simulink model "EstudioReguladores"  (R2024b)
settings: Solver=VariableStepAuto  StartTime=0.0  StopTime=50000  RelTol=1e-3
undefined symbols (not defined in the file): n, p1, p2, p3, Vi
libraries: slpidlib x32
(part 3 of 4)

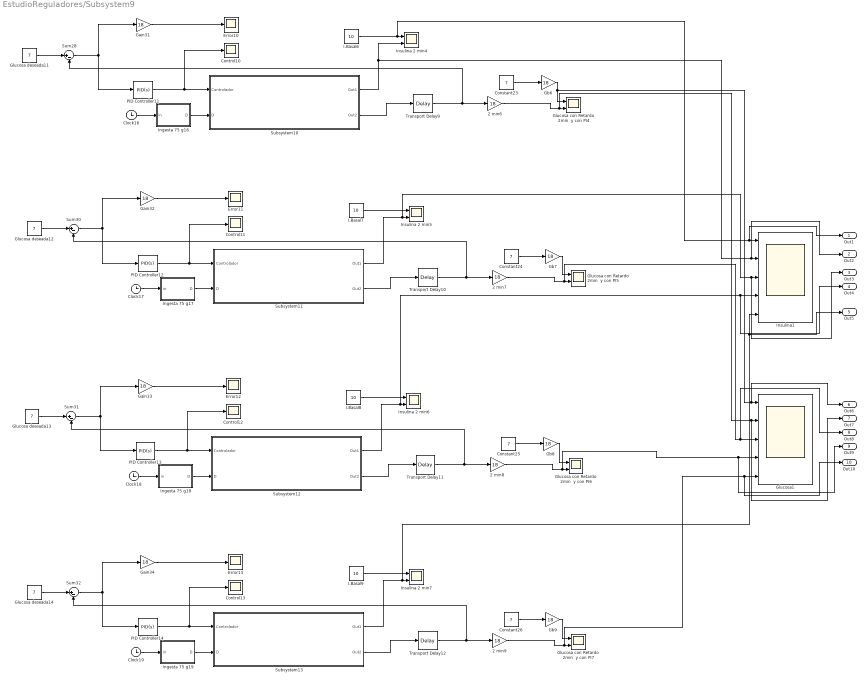
== system EstudioReguladores/Subsystem9 ==
  2 min{6..9} (4 alike) : Gain  Gain=18
  Clock{16..19} (4 alike) : Clock
  Constant{23..26} (4 alike) : Constant  Value=7
  Control{10..13} (4 alike) : Scope
  Error{10..13} (4 alike) : Scope
  Gain{31..34} (4 alike) : Gain  Gain=18
  Gb{6..9} (4 alike) : Gain  Gain=18
  Glucosa con Retardo 2min  y con PI{4..7} (4 alike) : Scope  NumInputPorts=2
  Glucosa deseada{11..14} (4 alike) : Constant  Value=7
  Glucosa1 : Scope  NumInputPorts=5
  I.Basal{6..9} (4 alike) : Constant  Value=10
  Ingesta 75 g16 : MATLAB Function  TreatAsAtomicUnit=on
  Ingesta 75 g17 : MATLAB Function  TreatAsAtomicUnit=on
  Ingesta 75 g18 : MATLAB Function  TreatAsAtomicUnit=on
  Ingesta 75 g19 : MATLAB Function  TreatAsAtomicUnit=on
  Insulina 2 min{4..7} (4 alike) : Scope  NumInputPorts=2
  Insulina1 : Scope  NumInputPorts=5
  PID Controller11 : slpidlib/PID Controller  Controller=PID  Form=Parallel  TimeDomain=Continuous-time  UseExternalTs=off  SampleTime=-1  IntegratorMethod=Forward Euler  FilterMethod=Forward Euler  ControllerParametersSource=internal  P=-0.3195  I=-0.3195/2998.95  UseKiTs=off  D=0  UseExternalDerivativeSource=off  N=10  UseFilter=on  TunerSelectOption=Transfer Function Based (PID Tuner App)  InitialConditionSource=internal  InitialConditionForIntegrator=0  InitialConditionForFilter=0  DifferentiatorICPrevScaledInput=0  ExternalReset=none  TrackingMode=off  Kt=1  LimitOutput=off  SatLimitsSource=internal  UpperSaturationLimit=inf  LowerSaturationLimit=-inf  LinearizeAsGain=on  AntiWindupMode=none  Kb=1  LimitIntegrator=off  UpperIntegratorSaturationLimit=inf  LowerIntegratorSaturationLimit=-inf  POutMin=[]  POutMax=[]  IOutMin=[]  IOutMax=[]  DOutMin=[]  DOutMax=[]  NOutMin=[]  NOutMax=[]  SumOutMin=[]  SumOutMax=[]  SaturationOutMin=[]  SaturationOutMax=[]  PParamMin=[]  PParamMax=[]  IParamMin=[]  IParamMax=[]  DParamMin=[]  DParamMax=[]  NParamMin=[]  NParamMax=[]  KbParamMin=[]  KbParamMax=[]  KtParamMin=[]  KtParamMax=[]  KbOutMin=[]  KbOutMax=[]  KtOutMin=[]  KtOutMax=[]  IntegratorOutMin=[]  IntegratorOutMax=[]  FilterOutMin=[]  FilterOutMax=[]  SumI1OutMin=[]  SumI1OutMax=[]  SumI2OutMin=[]  SumI2OutMax=[]  SumI3OutMin=[]  SumI3OutMax=[]  SumI4OutMin=[]  SumI4OutMax=[]  SumDOutMin=[]  SumDOutMax=[]  DifferentiatorOutMin=[]  DifferentiatorOutMax=[]  FilterDiffOutCoefMin=[]  FilterDiffOutCoefMax=[]  ReciprocalOutMin=[]  ReciprocalOutMax=[]  SumDenOutMin=[]  SumDenOutMax=[]  SumNumOutMin=[]  SumNumOutMax=[]  DivideOutMin=[]  DivideOutMax=[]  UdiffTsProdOutMin=[]  UdiffTsProdOutMax=[]  NTsProdOutMin=[]  NTsProdOutMax=[]  UintegralTsProdOutMin=[]  UintegralTsProdOutMax=[]  UngainTsProdOutMin=[]  UngainTsProdOutMax=[]  ClampingZeroOutDataTypeStr=Inherit: Inherit via back propagation  ClampingZeroOutMin=[]  ClampingZeroOutMax=[]  FilterDenConstantOutDataTypeStr=Inherit: Inherit via back propagation  FilterDenConstantOutMin=[]  FilterDenConstantOutMax=[]  PCopyOutDataTypeStr=Inherit: Inherit via back propagation  PCopyOutMin=[]  PCopyOutMax=[]  NCopyOutDataTypeStr=Inherit: Inherit via back propagation  NCopyOutMin=[]  NCopyOutMax=[]  IntegratorContinuousStateAttributes=''  IntegratorStateMustResolveToSignalObject=off  IntegratorRTWStateStorageClass=Auto  FilterContinuousStateAttributes=''  FilterStateMustResolveToSignalObject=off  FilterRTWStateStorageClass=Auto  ParallelPVariant=InternalParameters  IdealPVariant=Disabled  IVariant=InternalParameters  DVariant=InternalParameters  IntegratorVariant=Continuous  SatVariant=Disabled  AWVariant=Passthrough  PCopyVariant=Disabled  TRVariant=Disabled  FdbkBlocksVariant=Forward  IdealPFdbkVariant=Disabled  SatFdbkVariant=Disabled  DerivativeFilterVariant=ContFilter  NVariant=InternalParameters  NCopyVariant=Disabled  FilterICVariant=InternalICsFilter  IntegratorICVariant=InternalICs  ExternalResetVariant=Disabled  TRSumVariant=Passthrough  SumFdbkVariant=Disabled  SumVariant=Sum_PID  TsampFilterVariant=InternalTs  TsampNgainVariant=Passthrough  TsampIntegralVariant=Disabled_SignalSpec  ExternalSaturationOutDataTypeStr=Inherit: Same as second input  DerivativeSourceVariant=ErrorSignal  PreIntVariant=InternalPreInt
  PID Controller12 : slpidlib/PID Controller  Controller=PID  Form=Parallel  TimeDomain=Continuous-time  UseExternalTs=off  SampleTime=-1  IntegratorMethod=Forward Euler  FilterMethod=Forward Euler  ControllerParametersSource=internal  P=-0.3195  I=-0.3195/2998.95  UseKiTs=off  D=0.01  UseExternalDerivativeSource=off  N=10  UseFilter=on  TunerSelectOption=Transfer Function Based (PID Tuner App)  InitialConditionSource=internal  InitialConditionForIntegrator=0  InitialConditionForFilter=0  DifferentiatorICPrevScaledInput=0  ExternalReset=none  TrackingMode=off  Kt=1  LimitOutput=off  SatLimitsSource=internal  UpperSaturationLimit=inf  LowerSaturationLimit=-inf  LinearizeAsGain=on  AntiWindupMode=none  Kb=1  LimitIntegrator=off  UpperIntegratorSaturationLimit=inf  LowerIntegratorSaturationLimit=-inf  POutMin=[]  POutMax=[]  IOutMin=[]  IOutMax=[]  DOutMin=[]  DOutMax=[]  NOutMin=[]  NOutMax=[]  SumOutMin=[]  SumOutMax=[]  SaturationOutMin=[]  SaturationOutMax=[]  PParamMin=[]  PParamMax=[]  IParamMin=[]  IParamMax=[]  DParamMin=[]  DParamMax=[]  NParamMin=[]  NParamMax=[]  KbParamMin=[]  KbParamMax=[]  KtParamMin=[]  KtParamMax=[]  KbOutMin=[]  KbOutMax=[]  KtOutMin=[]  KtOutMax=[]  IntegratorOutMin=[]  IntegratorOutMax=[]  FilterOutMin=[]  FilterOutMax=[]  SumI1OutMin=[]  SumI1OutMax=[]  SumI2OutMin=[]  SumI2OutMax=[]  SumI3OutMin=[]  SumI3OutMax=[]  SumI4OutMin=[]  SumI4OutMax=[]  SumDOutMin=[]  SumDOutMax=[]  DifferentiatorOutMin=[]  DifferentiatorOutMax=[]  FilterDiffOutCoefMin=[]  FilterDiffOutCoefMax=[]  ReciprocalOutMin=[]  ReciprocalOutMax=[]  SumDenOutMin=[]  SumDenOutMax=[]  SumNumOutMin=[]  SumNumOutMax=[]  DivideOutMin=[]  DivideOutMax=[]  UdiffTsProdOutMin=[]  UdiffTsProdOutMax=[]  NTsProdOutMin=[]  NTsProdOutMax=[]  UintegralTsProdOutMin=[]  UintegralTsProdOutMax=[]  UngainTsProdOutMin=[]  UngainTsProdOutMax=[]  ClampingZeroOutDataTypeStr=Inherit: Inherit via back propagation  ClampingZeroOutMin=[]  ClampingZeroOutMax=[]  FilterDenConstantOutDataTypeStr=Inherit: Inherit via back propagation  FilterDenConstantOutMin=[]  FilterDenConstantOutMax=[]  PCopyOutDataTypeStr=Inherit: Inherit via back propagation  PCopyOutMin=[]  PCopyOutMax=[]  NCopyOutDataTypeStr=Inherit: Inherit via back propagation  NCopyOutMin=[]  NCopyOutMax=[]  IntegratorContinuousStateAttributes=''  IntegratorStateMustResolveToSignalObject=off  IntegratorRTWStateStorageClass=Auto  FilterContinuousStateAttributes=''  FilterStateMustResolveToSignalObject=off  FilterRTWStateStorageClass=Auto  ParallelPVariant=InternalParameters  IdealPVariant=Disabled  IVariant=InternalParameters  DVariant=InternalParameters  IntegratorVariant=Continuous  SatVariant=Disabled  AWVariant=Passthrough  PCopyVariant=Disabled  TRVariant=Disabled  FdbkBlocksVariant=Forward  IdealPFdbkVariant=Disabled  SatFdbkVariant=Disabled  DerivativeFilterVariant=ContFilter  NVariant=InternalParameters  NCopyVariant=Disabled  FilterICVariant=InternalICsFilter  IntegratorICVariant=InternalICs  ExternalResetVariant=Disabled  TRSumVariant=Passthrough  SumFdbkVariant=Disabled  SumVariant=Sum_PID  TsampFilterVariant=InternalTs  TsampNgainVariant=Passthrough  TsampIntegralVariant=Disabled_SignalSpec  ExternalSaturationOutDataTypeStr=Inherit: Same as second input  DerivativeSourceVariant=ErrorSignal  PreIntVariant=InternalPreInt
  PID Controller13 : slpidlib/PID Controller  Controller=PID  Form=Parallel  TimeDomain=Continuous-time  UseExternalTs=off  SampleTime=-1  IntegratorMethod=Forward Euler  FilterMethod=Forward Euler  ControllerParametersSource=internal  P=-0.3195  I=0  UseKiTs=off  D=0  UseExternalDerivativeSource=off  N=10  UseFilter=on  TunerSelectOption=Transfer Function Based (PID Tuner App)  InitialConditionSource=internal  InitialConditionForIntegrator=0  InitialConditionForFilter=0  DifferentiatorICPrevScaledInput=0  ExternalReset=none  TrackingMode=off  Kt=1  LimitOutput=off  SatLimitsSource=internal  UpperSaturationLimit=inf  LowerSaturationLimit=-inf  LinearizeAsGain=on  AntiWindupMode=none  Kb=1  LimitIntegrator=off  UpperIntegratorSaturationLimit=inf  LowerIntegratorSaturationLimit=-inf  POutMin=[]  POutMax=[]  IOutMin=[]  IOutMax=[]  DOutMin=[]  DOutMax=[]  NOutMin=[]  NOutMax=[]  SumOutMin=[]  SumOutMax=[]  SaturationOutMin=[]  SaturationOutMax=[]  PParamMin=[]  PParamMax=[]  IParamMin=[]  IParamMax=[]  DParamMin=[]  DParamMax=[]  NParamMin=[]  NParamMax=[]  KbParamMin=[]  KbParamMax=[]  KtParamMin=[]  KtParamMax=[]  KbOutMin=[]  KbOutMax=[]  KtOutMin=[]  KtOutMax=[]  IntegratorOutMin=[]  IntegratorOutMax=[]  FilterOutMin=[]  FilterOutMax=[]  SumI1OutMin=[]  SumI1OutMax=[]  SumI2OutMin=[]  SumI2OutMax=[]  SumI3OutMin=[]  SumI3OutMax=[]  SumI4OutMin=[]  SumI4OutMax=[]  SumDOutMin=[]  SumDOutMax=[]  DifferentiatorOutMin=[]  DifferentiatorOutMax=[]  FilterDiffOutCoefMin=[]  FilterDiffOutCoefMax=[]  ReciprocalOutMin=[]  ReciprocalOutMax=[]  SumDenOutMin=[]  SumDenOutMax=[]  SumNumOutMin=[]  SumNumOutMax=[]  DivideOutMin=[]  DivideOutMax=[]  UdiffTsProdOutMin=[]  UdiffTsProdOutMax=[]  NTsProdOutMin=[]  NTsProdOutMax=[]  UintegralTsProdOutMin=[]  UintegralTsProdOutMax=[]  UngainTsProdOutMin=[]  UngainTsProdOutMax=[]  ClampingZeroOutDataTypeStr=Inherit: Inherit via back propagation  ClampingZeroOutMin=[]  ClampingZeroOutMax=[]  FilterDenConstantOutDataTypeStr=Inherit: Inherit via back propagation  FilterDenConstantOutMin=[]  FilterDenConstantOutMax=[]  PCopyOutDataTypeStr=Inherit: Inherit via back propagation  PCopyOutMin=[]  PCopyOutMax=[]  NCopyOutDataTypeStr=Inherit: Inherit via back propagation  NCopyOutMin=[]  NCopyOutMax=[]  IntegratorContinuousStateAttributes=''  IntegratorStateMustResolveToSignalObject=off  IntegratorRTWStateStorageClass=Auto  FilterContinuousStateAttributes=''  FilterStateMustResolveToSignalObject=off  FilterRTWStateStorageClass=Auto  ParallelPVariant=InternalParameters  IdealPVariant=Disabled  IVariant=InternalParameters  DVariant=InternalParameters  IntegratorVariant=Continuous  SatVariant=Disabled  AWVariant=Passthrough  PCopyVariant=Disabled  TRVariant=Disabled  FdbkBlocksVariant=Forward  IdealPFdbkVariant=Disabled  SatFdbkVariant=Disabled  DerivativeFilterVariant=ContFilter  NVariant=InternalParameters  NCopyVariant=Disabled  FilterICVariant=InternalICsFilter  IntegratorICVariant=InternalICs  ExternalResetVariant=Disabled  TRSumVariant=Passthrough  SumFdbkVariant=Disabled  SumVariant=Sum_PID  TsampFilterVariant=InternalTs  TsampNgainVariant=Passthrough  TsampIntegralVariant=Disabled_SignalSpec  ExternalSaturationOutDataTypeStr=Inherit: Same as second input  DerivativeSourceVariant=ErrorSignal  PreIntVariant=InternalPreInt
  PID Controller14 : slpidlib/PID Controller  Controller=PID  Form=Parallel  TimeDomain=Continuous-time  UseExternalTs=off  SampleTime=-1  IntegratorMethod=Forward Euler  FilterMethod=Forward Euler  ControllerParametersSource=internal  P=-0.3195  I=0  UseKiTs=off  D=0.01  UseExternalDerivativeSource=off  N=10  UseFilter=on  TunerSelectOption=Transfer Function Based (PID Tuner App)  InitialConditionSource=internal  InitialConditionForIntegrator=0  InitialConditionForFilter=0  DifferentiatorICPrevScaledInput=0  ExternalReset=none  TrackingMode=off  Kt=1  LimitOutput=off  SatLimitsSource=internal  UpperSaturationLimit=inf  LowerSaturationLimit=-inf  LinearizeAsGain=on  AntiWindupMode=none  Kb=1  LimitIntegrator=off  UpperIntegratorSaturationLimit=inf  LowerIntegratorSaturationLimit=-inf  POutMin=[]  POutMax=[]  IOutMin=[]  IOutMax=[]  DOutMin=[]  DOutMax=[]  NOutMin=[]  NOutMax=[]  SumOutMin=[]  SumOutMax=[]  SaturationOutMin=[]  SaturationOutMax=[]  PParamMin=[]  PParamMax=[]  IParamMin=[]  IParamMax=[]  DParamMin=[]  DParamMax=[]  NParamMin=[]  NParamMax=[]  KbParamMin=[]  KbParamMax=[]  KtParamMin=[]  KtParamMax=[]  KbOutMin=[]  KbOutMax=[]  KtOutMin=[]  KtOutMax=[]  IntegratorOutMin=[]  IntegratorOutMax=[]  FilterOutMin=[]  FilterOutMax=[]  SumI1OutMin=[]  SumI1OutMax=[]  SumI2OutMin=[]  SumI2OutMax=[]  SumI3OutMin=[]  SumI3OutMax=[]  SumI4OutMin=[]  SumI4OutMax=[]  SumDOutMin=[]  SumDOutMax=[]  DifferentiatorOutMin=[]  DifferentiatorOutMax=[]  FilterDiffOutCoefMin=[]  FilterDiffOutCoefMax=[]  ReciprocalOutMin=[]  ReciprocalOutMax=[]  SumDenOutMin=[]  SumDenOutMax=[]  SumNumOutMin=[]  SumNumOutMax=[]  DivideOutMin=[]  DivideOutMax=[]  UdiffTsProdOutMin=[]  UdiffTsProdOutMax=[]  NTsProdOutMin=[]  NTsProdOutMax=[]  UintegralTsProdOutMin=[]  UintegralTsProdOutMax=[]  UngainTsProdOutMin=[]  UngainTsProdOutMax=[]  ClampingZeroOutDataTypeStr=Inherit: Inherit via back propagation  ClampingZeroOutMin=[]  ClampingZeroOutMax=[]  FilterDenConstantOutDataTypeStr=Inherit: Inherit via back propagation  FilterDenConstantOutMin=[]  FilterDenConstantOutMax=[]  PCopyOutDataTypeStr=Inherit: Inherit via back propagation  PCopyOutMin=[]  PCopyOutMax=[]  NCopyOutDataTypeStr=Inherit: Inherit via back propagation  NCopyOutMin=[]  NCopyOutMax=[]  IntegratorContinuousStateAttributes=''  IntegratorStateMustResolveToSignalObject=off  IntegratorRTWStateStorageClass=Auto  FilterContinuousStateAttributes=''  FilterStateMustResolveToSignalObject=off  FilterRTWStateStorageClass=Auto  ParallelPVariant=InternalParameters  IdealPVariant=Disabled  IVariant=InternalParameters  DVariant=InternalParameters  IntegratorVariant=Continuous  SatVariant=Disabled  AWVariant=Passthrough  PCopyVariant=Disabled  TRVariant=Disabled  FdbkBlocksVariant=Forward  IdealPFdbkVariant=Disabled  SatFdbkVariant=Disabled  DerivativeFilterVariant=ContFilter  NVariant=InternalParameters  NCopyVariant=Disabled  FilterICVariant=InternalICsFilter  IntegratorICVariant=InternalICs  ExternalResetVariant=Disabled  TRSumVariant=Passthrough  SumFdbkVariant=Disabled  SumVariant=Sum_PID  TsampFilterVariant=InternalTs  TsampNgainVariant=Passthrough  TsampIntegralVariant=Disabled_SignalSpec  ExternalSaturationOutDataTypeStr=Inherit: Same as second input  DerivativeSourceVariant=ErrorSignal  PreIntVariant=InternalPreInt
  Subsystem10 : Subsystem
  Subsystem11 : Subsystem
  Subsystem12 : Subsystem
  Subsystem13 : Subsystem
  Sum{28,30..32} (4 alike) : Sum  Inputs=|+-
  Transport Delay{9..12} (4 alike) : TransportDelay  DelayTime=600  InitialOutput=7
  Out1 : Outport
  Out2 : Outport  Port=2
  Out3 : Outport  Port=3
  Out4 : Outport  Port=4
  Out5 : Outport  Port=5
  Out6 : Outport  Port=6
  Out7 : Outport  Port=7
  Out8 : Outport  Port=8
  Out9 : Outport  Port=9
  Out10 : Outport  Port=10
  wires:
  Glucosa deseada13/1 -> Sum31/1
  Subsystem12/1(Out1) -> Out4/1, Insulina1/4, Insulina 2 min6/2
  2 min9/1 -> Out10/1, Glucosa1/5, Glucosa con Retardo 2min  y con PI7/2
  I.Basal6/1 -> Out1/1, Insulina1/1, Insulina 2 min4/1
  Transport Delay12/1 -> Sum32/2, 2 min9/1
  Glucosa deseada14/1 -> Sum32/1
  Gain31/1 -> Error10/1
  I.Basal9/1 -> Insulina 2 min7/1
  PID Controller13/1 -> Control12/1, Subsystem12/1(Controlador)
  Glucosa deseada11/1 -> Sum28/1
  I.Basal8/1 -> Insulina 2 min6/1
  Ingesta 75 g19/1(D) -> Subsystem13/2(D)
  Gb8/1 -> Glucosa con Retardo 2min  y con PI6/1
  2 min8/1 -> Out9/1, Glucosa1/4, Glucosa con Retardo 2min  y con PI6/2
  PID Controller12/1 -> Control11/1, Subsystem11/1(Controlador)
  Gb9/1 -> Glucosa con Retardo 2min  y con PI7/1
  Sum32/1 -> PID Controller14/1, Gain34/1
  Gb6/1 -> Out6/1, Glucosa1/1, Glucosa con Retardo 2min  y con PI4/1
  Transport Delay11/1 -> Sum31/2, 2 min8/1
  Clock18/1 -> Ingesta 75 g18/1(in)
  PID Controller14/1 -> Control13/1, Subsystem13/1(Controlador)
  Subsystem10/1(Out1) -> Insulina 2 min4/2, Out2/1, Insulina1/2
  PID Controller11/1 -> Control10/1, Subsystem10/1(Controlador)
  2 min6/1 -> Out7/1, Glucosa1/2, Glucosa con Retardo 2min  y con PI4/2
  Subsystem12/2(Out2) -> Transport Delay11/1
  Gb7/1 -> Glucosa con Retardo 2min  y con PI5/1
  Subsystem13/1(Out1) -> Out5/1, Insulina1/5, Insulina 2 min7/2
  Sum31/1 -> PID Controller13/1, Gain33/1
  2 min7/1 -> Out8/1, Glucosa1/3, Glucosa con Retardo 2min  y con PI5/2
  Subsystem13/2(Out2) -> Transport Delay12/1
  Gain33/1 -> Error12/1
  Transport Delay9/1 -> Sum28/2, 2 min6/1
  Constant25/1 -> Gb8/1
  Ingesta 75 g17/1(D) -> Subsystem11/2(D)
  Ingesta 75 g18/1(D) -> Subsystem12/2(D)
  Gain34/1 -> Error13/1
  Clock19/1 -> Ingesta 75 g19/1(in)
  Glucosa deseada12/1 -> Sum30/1
  Constant26/1 -> Gb9/1
  Ingesta 75 g16/1(D) -> Subsystem10/2(D)
  Subsystem11/1(Out1) -> Out3/1, Insulina1/3, Insulina 2 min5/2
  Sum28/1 -> PID Controller11/1, Gain31/1
  Constant23/1 -> Gb6/1
  Sum30/1 -> PID Controller12/1, Gain32/1
  Transport Delay10/1 -> Sum30/2, 2 min7/1
  I.Basal7/1 -> Insulina 2 min5/1
  Subsystem11/2(Out2) -> Transport Delay10/1
  Clock17/1 -> Ingesta 75 g17/1(in)
  Subsystem10/2(Out2) -> Transport Delay9/1
  Constant24/1 -> Gb7/1
  Gain32/1 -> Error11/1
  Clock16/1 -> Ingesta 75 g16/1(in)

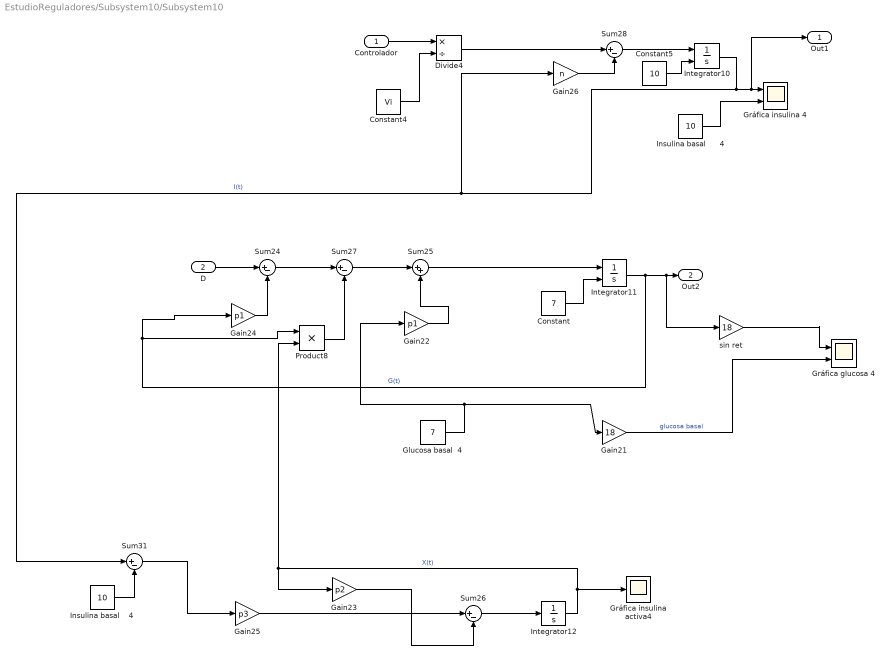
== system EstudioReguladores/Subsystem10/Subsystem10 ==
  Controlador : Inport
  D : Inport  Port=2
  Constant : Constant  Value=7
  Constant4 : Constant  Value=Vi
  Constant5 : Constant  Value=10
  Divide4 : Product  Inputs=*/
  Gain21 : Gain  Gain=18
  Gain22 : Gain  Gain=p1
  Gain23 : Gain  Gain=p2
  Gain24 : Gain  Gain=p1
  Gain25 : Gain  Gain=p3
  Gain26 : Gain  Gain=n
  Glucosa basal  4 : Constant  Value=7
  Gráfica glucosa 4 : Scope  NumInputPorts=2
  Gráfica insulina 4 : Scope  NumInputPorts=2
  Gráfica insulina activa4 : Scope
  Insulina basal      4 : Constant  Value=10
  Insulina basal    4 : Constant  Value=10
  Integrator10 : Integrator  InitialConditionSource=external
  Integrator11 : Integrator  InitialConditionSource=external  InitialCondition=7
  Integrator12 : Integrator
  Product8 : Product
  Sum{24,26..28,31} (5 alike) : Sum  Inputs=|+-
  Sum25 : Sum  Inputs=|++
  sin ret : Gain  Gain=18
  Out1 : Outport
  Out2 : Outport  Port=2
  wires:
  Gain26/1 -> Sum28/2
  Glucosa basal  4/1 -> Gain22/1, Gain21/1
  D/1 -> Sum24/1
  Gain21/1 -> Gráfica glucosa 4/2  "glucosa basal"
  Integrator11/1 -> sin ret/1, Out2/1, Gain24/1, Product8/1  "G(t)"
  Integrator12/1 -> Product8/2, Gain23/1, Gráfica insulina activa4/1  "X(t)"
  Gain25/1 -> Sum26/1
  Integrator10/1 -> Out1/1, Gráfica insulina 4/1, Sum31/1, Gain26/1  "I(t)"
  Constant5/1 -> Integrator10/2
  Sum31/1 -> Gain25/1
  Sum26/1 -> Integrator12/1
  Gain23/1 -> Sum26/2
  Sum28/1 -> Integrator10/1
  Sum24/1 -> Sum27/1
  Sum25/1 -> Integrator11/1
  Gain24/1 -> Sum24/2
  Insulina basal      4/1 -> Gráfica insulina 4/2
  Sum27/1 -> Sum25/1
  Insulina basal    4/1 -> Sum31/2
  Divide4/1 -> Sum28/1
  Gain22/1 -> Sum25/2
  Product8/1 -> Sum27/2
  Constant4/1 -> Divide4/2
  Constant/1 -> Integrator11/2
  Controlador/1 -> Divide4/1
  sin ret/1 -> Gráfica glucosa 4/1

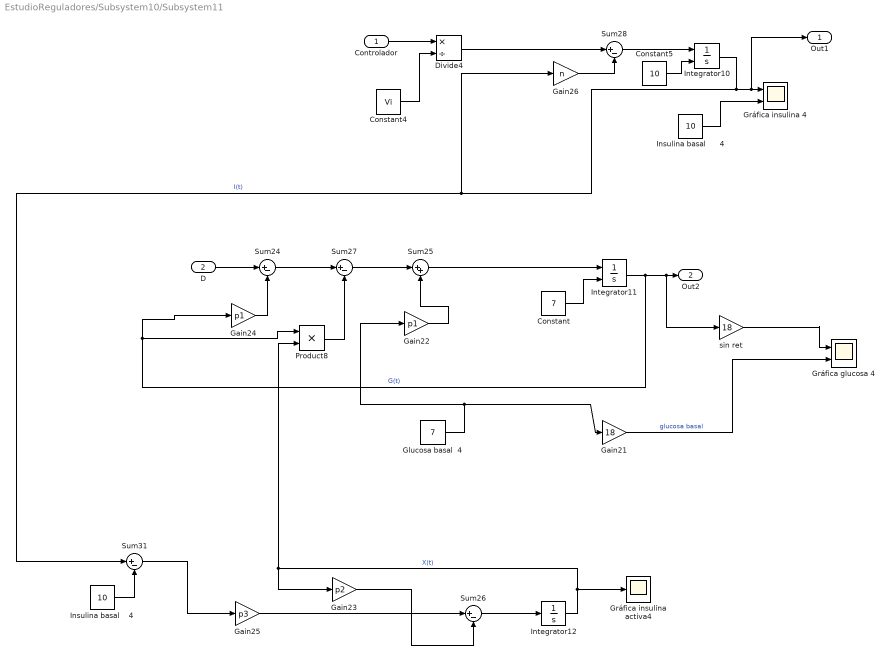
== system EstudioReguladores/Subsystem10/Subsystem11 ==
  Controlador : Inport
  D : Inport  Port=2
  Constant : Constant  Value=7
  Constant4 : Constant  Value=Vi
  Constant5 : Constant  Value=10
  Divide4 : Product  Inputs=*/
  Gain21 : Gain  Gain=18
  Gain22 : Gain  Gain=p1
  Gain23 : Gain  Gain=p2
  Gain24 : Gain  Gain=p1
  Gain25 : Gain  Gain=p3
  Gain26 : Gain  Gain=n
  Glucosa basal  4 : Constant  Value=7
  Gráfica glucosa 4 : Scope  NumInputPorts=2
  Gráfica insulina 4 : Scope  NumInputPorts=2
  Gráfica insulina activa4 : Scope
  Insulina basal      4 : Constant  Value=10
  Insulina basal    4 : Constant  Value=10
  Integrator10 : Integrator  InitialConditionSource=external
  Integrator11 : Integrator  InitialConditionSource=external  InitialCondition=7
  Integrator12 : Integrator
  Product8 : Product
  Sum{24,26..28,31} (5 alike) : Sum  Inputs=|+-
  Sum25 : Sum  Inputs=|++
  sin ret : Gain  Gain=18
  Out1 : Outport
  Out2 : Outport  Port=2
  wires:
  Gain26/1 -> Sum28/2
  Glucosa basal  4/1 -> Gain22/1, Gain21/1
  D/1 -> Sum24/1
  Gain21/1 -> Gráfica glucosa 4/2  "glucosa basal"
  Integrator11/1 -> sin ret/1, Out2/1, Gain24/1, Product8/1  "G(t)"
  Integrator12/1 -> Product8/2, Gain23/1, Gráfica insulina activa4/1  "X(t)"
  Gain25/1 -> Sum26/1
  Integrator10/1 -> Out1/1, Gráfica insulina 4/1, Sum31/1, Gain26/1  "I(t)"
  Constant5/1 -> Integrator10/2
  Sum31/1 -> Gain25/1
  Sum26/1 -> Integrator12/1
  Gain23/1 -> Sum26/2
  Sum28/1 -> Integrator10/1
  Sum24/1 -> Sum27/1
  Sum25/1 -> Integrator11/1
  Gain24/1 -> Sum24/2
  Insulina basal      4/1 -> Gráfica insulina 4/2
  Sum27/1 -> Sum25/1
  Insulina basal    4/1 -> Sum31/2
  Divide4/1 -> Sum28/1
  Gain22/1 -> Sum25/2
  Product8/1 -> Sum27/2
  Constant4/1 -> Divide4/2
  Constant/1 -> Integrator11/2
  Controlador/1 -> Divide4/1
  sin ret/1 -> Gráfica glucosa 4/1

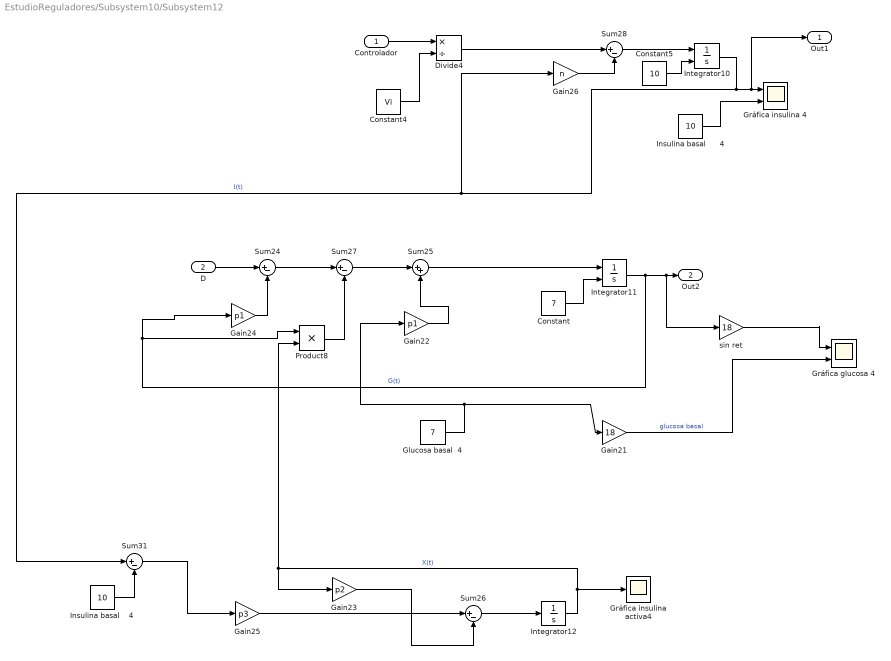
== system EstudioReguladores/Subsystem10/Subsystem12 ==
  Controlador : Inport
  D : Inport  Port=2
  Constant : Constant  Value=7
  Constant4 : Constant  Value=Vi
  Constant5 : Constant  Value=10
  Divide4 : Product  Inputs=*/
  Gain21 : Gain  Gain=18
  Gain22 : Gain  Gain=p1
  Gain23 : Gain  Gain=p2
  Gain24 : Gain  Gain=p1
  Gain25 : Gain  Gain=p3
  Gain26 : Gain  Gain=n
  Glucosa basal  4 : Constant  Value=7
  Gráfica glucosa 4 : Scope  NumInputPorts=2
  Gráfica insulina 4 : Scope  NumInputPorts=2
  Gráfica insulina activa4 : Scope
  Insulina basal      4 : Constant  Value=10
  Insulina basal    4 : Constant  Value=10
  Integrator10 : Integrator  InitialConditionSource=external
  Integrator11 : Integrator  InitialConditionSource=external  InitialCondition=7
  Integrator12 : Integrator
  Product8 : Product
  Sum{24,26..28,31} (5 alike) : Sum  Inputs=|+-
  Sum25 : Sum  Inputs=|++
  sin ret : Gain  Gain=18
  Out1 : Outport
  Out2 : Outport  Port=2
  wires:
  Gain26/1 -> Sum28/2
  Glucosa basal  4/1 -> Gain22/1, Gain21/1
  D/1 -> Sum24/1
  Gain21/1 -> Gráfica glucosa 4/2  "glucosa basal"
  Integrator11/1 -> sin ret/1, Out2/1, Gain24/1, Product8/1  "G(t)"
  Integrator12/1 -> Product8/2, Gain23/1, Gráfica insulina activa4/1  "X(t)"
  Gain25/1 -> Sum26/1
  Integrator10/1 -> Out1/1, Gráfica insulina 4/1, Sum31/1, Gain26/1  "I(t)"
  Constant5/1 -> Integrator10/2
  Sum31/1 -> Gain25/1
  Sum26/1 -> Integrator12/1
  Gain23/1 -> Sum26/2
  Sum28/1 -> Integrator10/1
  Sum24/1 -> Sum27/1
  Sum25/1 -> Integrator11/1
  Gain24/1 -> Sum24/2
  Insulina basal      4/1 -> Gráfica insulina 4/2
  Sum27/1 -> Sum25/1
  Insulina basal    4/1 -> Sum31/2
  Divide4/1 -> Sum28/1
  Gain22/1 -> Sum25/2
  Product8/1 -> Sum27/2
  Constant4/1 -> Divide4/2
  Constant/1 -> Integrator11/2
  Controlador/1 -> Divide4/1
  sin ret/1 -> Gráfica glucosa 4/1

== system EstudioReguladores/Subsystem10/Subsystem13 ==
  Controlador : Inport
  D : Inport  Port=2
  Constant : Constant  Value=7
  Constant4 : Constant  Value=Vi
  Constant5 : Constant  Value=10
  Divide4 : Product  Inputs=*/
  Gain21 : Gain  Gain=18
  Gain22 : Gain  Gain=p1
  Gain23 : Gain  Gain=p2
  Gain24 : Gain  Gain=p1
  Gain25 : Gain  Gain=p3
  Gain26 : Gain  Gain=n
  Glucosa basal  4 : Constant  Value=7
  Gráfica glucosa 4 : Scope  NumInputPorts=2
  Gráfica insulina 4 : Scope  NumInputPorts=2
  Gráfica insulina activa4 : Scope
  Insulina basal      4 : Constant  Value=10
  Insulina basal    4 : Constant  Value=10
  Integrator10 : Integrator  InitialConditionSource=external
  Integrator11 : Integrator  InitialConditionSource=external  InitialCondition=7
  Integrator12 : Integrator
  Product8 : Product
  Sum{24,26..28,31} (5 alike) : Sum  Inputs=|+-
  Sum25 : Sum  Inputs=|++
  sin ret : Gain  Gain=18
  Out1 : Outport
  Out2 : Outport  Port=2
  wires:
  Gain26/1 -> Sum28/2
  Glucosa basal  4/1 -> Gain22/1, Gain21/1
  D/1 -> Sum24/1
  Gain21/1 -> Gráfica glucosa 4/2  "glucosa basal"
  Integrator11/1 -> sin ret/1, Out2/1, Gain24/1, Product8/1  "G(t)"
  Integrator12/1 -> Product8/2, Gain23/1, Gráfica insulina activa4/1  "X(t)"
  Gain25/1 -> Sum26/1
  Integrator10/1 -> Out1/1, Gráfica insulina 4/1, Sum31/1, Gain26/1  "I(t)"
  Constant5/1 -> Integrator10/2
  Sum31/1 -> Gain25/1
  Sum26/1 -> Integrator12/1
  Gain23/1 -> Sum26/2
  Sum28/1 -> Integrator10/1
  Sum24/1 -> Sum27/1
  Sum25/1 -> Integrator11/1
  Gain24/1 -> Sum24/2
  Insulina basal      4/1 -> Gráfica insulina 4/2
  Sum27/1 -> Sum25/1
  Insulina basal    4/1 -> Sum31/2
  Divide4/1 -> Sum28/1
  Gain22/1 -> Sum25/2
  Product8/1 -> Sum27/2
  Constant4/1 -> Divide4/2
  Constant/1 -> Integrator11/2
  Controlador/1 -> Divide4/1
  sin ret/1 -> Gráfica glucosa 4/1

== system EstudioReguladores/Subsystem11/Subsystem10 ==
  Controlador : Inport
  D : Inport  Port=2
  Constant : Constant  Value=7
  Constant4 : Constant  Value=Vi
  Constant5 : Constant  Value=10
  Divide4 : Product  Inputs=*/
  Gain21 : Gain  Gain=18
  Gain22 : Gain  Gain=p1
  Gain23 : Gain  Gain=p2
  Gain24 : Gain  Gain=p1
  Gain25 : Gain  Gain=p3
  Gain26 : Gain  Gain=n
  Glucosa basal  4 : Constant  Value=7
  Gráfica glucosa 4 : Scope  NumInputPorts=2
  Gráfica insulina 4 : Scope  NumInputPorts=2
  Gráfica insulina activa4 : Scope
  Insulina basal      4 : Constant  Value=10
  Insulina basal    4 : Constant  Value=10
  Integrator10 : Integrator  InitialConditionSource=external
  Integrator11 : Integrator  InitialConditionSource=external  InitialCondition=7
  Integrator12 : Integrator
  Product8 : Product
  Sum{24,26..28,31} (5 alike) : Sum  Inputs=|+-
  Sum25 : Sum  Inputs=|++
  sin ret : Gain  Gain=18
  Out1 : Outport
  Out2 : Outport  Port=2
  wires:
  Gain26/1 -> Sum28/2
  Glucosa basal  4/1 -> Gain22/1, Gain21/1
  D/1 -> Sum24/1
  Gain21/1 -> Gráfica glucosa 4/2  "glucosa basal"
  Integrator11/1 -> sin ret/1, Out2/1, Gain24/1, Product8/1  "G(t)"
  Integrator12/1 -> Product8/2, Gain23/1, Gráfica insulina activa4/1  "X(t)"
  Gain25/1 -> Sum26/1
  Integrator10/1 -> Out1/1, Gráfica insulina 4/1, Sum31/1, Gain26/1  "I(t)"
  Constant5/1 -> Integrator10/2
  Sum31/1 -> Gain25/1
  Sum26/1 -> Integrator12/1
  Gain23/1 -> Sum26/2
  Sum28/1 -> Integrator10/1
  Sum24/1 -> Sum27/1
  Sum25/1 -> Integrator11/1
  Gain24/1 -> Sum24/2
  Insulina basal      4/1 -> Gráfica insulina 4/2
  Sum27/1 -> Sum25/1
  Insulina basal    4/1 -> Sum31/2
  Divide4/1 -> Sum28/1
  Gain22/1 -> Sum25/2
  Product8/1 -> Sum27/2
  Constant4/1 -> Divide4/2
  Constant/1 -> Integrator11/2
  Controlador/1 -> Divide4/1
  sin ret/1 -> Gráfica glucosa 4/1

== system EstudioReguladores/Subsystem11/Subsystem11 ==
  Controlador : Inport
  D : Inport  Port=2
  Constant : Constant  Value=7
  Constant4 : Constant  Value=Vi
  Constant5 : Constant  Value=10
  Divide4 : Product  Inputs=*/
  Gain21 : Gain  Gain=18
  Gain22 : Gain  Gain=p1
  Gain23 : Gain  Gain=p2
  Gain24 : Gain  Gain=p1
  Gain25 : Gain  Gain=p3
  Gain26 : Gain  Gain=n
  Glucosa basal  4 : Constant  Value=7
  Gráfica glucosa 4 : Scope  NumInputPorts=2
  Gráfica insulina 4 : Scope  NumInputPorts=2
  Gráfica insulina activa4 : Scope
  Insulina basal      4 : Constant  Value=10
  Insulina basal    4 : Constant  Value=10
  Integrator10 : Integrator  InitialConditionSource=external
  Integrator11 : Integrator  InitialConditionSource=external  InitialCondition=7
  Integrator12 : Integrator
  Product8 : Product
  Sum{24,26..28,31} (5 alike) : Sum  Inputs=|+-
  Sum25 : Sum  Inputs=|++
  sin ret : Gain  Gain=18
  Out1 : Outport
  Out2 : Outport  Port=2
  wires:
  Gain26/1 -> Sum28/2
  Glucosa basal  4/1 -> Gain22/1, Gain21/1
  D/1 -> Sum24/1
  Gain21/1 -> Gráfica glucosa 4/2  "glucosa basal"
  Integrator11/1 -> sin ret/1, Out2/1, Gain24/1, Product8/1  "G(t)"
  Integrator12/1 -> Product8/2, Gain23/1, Gráfica insulina activa4/1  "X(t)"
  Gain25/1 -> Sum26/1
  Integrator10/1 -> Out1/1, Gráfica insulina 4/1, Sum31/1, Gain26/1  "I(t)"
  Constant5/1 -> Integrator10/2
  Sum31/1 -> Gain25/1
  Sum26/1 -> Integrator12/1
  Gain23/1 -> Sum26/2
  Sum28/1 -> Integrator10/1
  Sum24/1 -> Sum27/1
  Sum25/1 -> Integrator11/1
  Gain24/1 -> Sum24/2
  Insulina basal      4/1 -> Gráfica insulina 4/2
  Sum27/1 -> Sum25/1
  Insulina basal    4/1 -> Sum31/2
  Divide4/1 -> Sum28/1
  Gain22/1 -> Sum25/2
  Product8/1 -> Sum27/2
  Constant4/1 -> Divide4/2
  Constant/1 -> Integrator11/2
  Controlador/1 -> Divide4/1
  sin ret/1 -> Gráfica glucosa 4/1

== system EstudioReguladores/Subsystem11/Subsystem12 ==
  Controlador : Inport
  D : Inport  Port=2
  Constant : Constant  Value=7
  Constant4 : Constant  Value=Vi
  Constant5 : Constant  Value=10
  Divide4 : Product  Inputs=*/
  Gain21 : Gain  Gain=18
  Gain22 : Gain  Gain=p1
  Gain23 : Gain  Gain=p2
  Gain24 : Gain  Gain=p1
  Gain25 : Gain  Gain=p3
  Gain26 : Gain  Gain=n
  Glucosa basal  4 : Constant  Value=7
  Gráfica glucosa 4 : Scope  NumInputPorts=2
  Gráfica insulina 4 : Scope  NumInputPorts=2
  Gráfica insulina activa4 : Scope
  Insulina basal      4 : Constant  Value=10
  Insulina basal    4 : Constant  Value=10
  Integrator10 : Integrator  InitialConditionSource=external
  Integrator11 : Integrator  InitialConditionSource=external  InitialCondition=7
  Integrator12 : Integrator
  Product8 : Product
  Sum{24,26..28,31} (5 alike) : Sum  Inputs=|+-
  Sum25 : Sum  Inputs=|++
  sin ret : Gain  Gain=18
  Out1 : Outport
  Out2 : Outport  Port=2
  wires:
  Gain26/1 -> Sum28/2
  Glucosa basal  4/1 -> Gain22/1, Gain21/1
  D/1 -> Sum24/1
  Gain21/1 -> Gráfica glucosa 4/2  "glucosa basal"
  Integrator11/1 -> sin ret/1, Out2/1, Gain24/1, Product8/1  "G(t)"
  Integrator12/1 -> Product8/2, Gain23/1, Gráfica insulina activa4/1  "X(t)"
  Gain25/1 -> Sum26/1
  Integrator10/1 -> Out1/1, Gráfica insulina 4/1, Sum31/1, Gain26/1  "I(t)"
  Constant5/1 -> Integrator10/2
  Sum31/1 -> Gain25/1
  Sum26/1 -> Integrator12/1
  Gain23/1 -> Sum26/2
  Sum28/1 -> Integrator10/1
  Sum24/1 -> Sum27/1
  Sum25/1 -> Integrator11/1
  Gain24/1 -> Sum24/2
  Insulina basal      4/1 -> Gráfica insulina 4/2
  Sum27/1 -> Sum25/1
  Insulina basal    4/1 -> Sum31/2
  Divide4/1 -> Sum28/1
  Gain22/1 -> Sum25/2
  Product8/1 -> Sum27/2
  Constant4/1 -> Divide4/2
  Constant/1 -> Integrator11/2
  Controlador/1 -> Divide4/1
  sin ret/1 -> Gráfica glucosa 4/1

== system EstudioReguladores/Subsystem11/Subsystem13 ==
  Controlador : Inport
  D : Inport  Port=2
  Constant : Constant  Value=7
  Constant4 : Constant  Value=Vi
  Constant5 : Constant  Value=10
  Divide4 : Product  Inputs=*/
  Gain21 : Gain  Gain=18
  Gain22 : Gain  Gain=p1
  Gain23 : Gain  Gain=p2
  Gain24 : Gain  Gain=p1
  Gain25 : Gain  Gain=p3
  Gain26 : Gain  Gain=n
  Glucosa basal  4 : Constant  Value=7
  Gráfica glucosa 4 : Scope  NumInputPorts=2
  Gráfica insulina 4 : Scope  NumInputPorts=2
  Gráfica insulina activa4 : Scope
  Insulina basal      4 : Constant  Value=10
  Insulina basal    4 : Constant  Value=10
  Integrator10 : Integrator  InitialConditionSource=external
  Integrator11 : Integrator  InitialConditionSource=external  InitialCondition=7
  Integrator12 : Integrator
  Product8 : Product
  Sum{24,26..28,31} (5 alike) : Sum  Inputs=|+-
  Sum25 : Sum  Inputs=|++
  sin ret : Gain  Gain=18
  Out1 : Outport
  Out2 : Outport  Port=2
  wires:
  Gain26/1 -> Sum28/2
  Glucosa basal  4/1 -> Gain22/1, Gain21/1
  D/1 -> Sum24/1
  Gain21/1 -> Gráfica glucosa 4/2  "glucosa basal"
  Integrator11/1 -> sin ret/1, Out2/1, Gain24/1, Product8/1  "G(t)"
  Integrator12/1 -> Product8/2, Gain23/1, Gráfica insulina activa4/1  "X(t)"
  Gain25/1 -> Sum26/1
  Integrator10/1 -> Out1/1, Gráfica insulina 4/1, Sum31/1, Gain26/1  "I(t)"
  Constant5/1 -> Integrator10/2
  Sum31/1 -> Gain25/1
  Sum26/1 -> Integrator12/1
  Gain23/1 -> Sum26/2
  Sum28/1 -> Integrator10/1
  Sum24/1 -> Sum27/1
  Sum25/1 -> Integrator11/1
  Gain24/1 -> Sum24/2
  Insulina basal      4/1 -> Gráfica insulina 4/2
  Sum27/1 -> Sum25/1
  Insulina basal    4/1 -> Sum31/2
  Divide4/1 -> Sum28/1
  Gain22/1 -> Sum25/2
  Product8/1 -> Sum27/2
  Constant4/1 -> Divide4/2
  Constant/1 -> Integrator11/2
  Controlador/1 -> Divide4/1
  sin ret/1 -> Gráfica glucosa 4/1

== system EstudioReguladores/Subsystem12/Subsystem10 ==
  Controlador : Inport
  D : Inport  Port=2
  Constant : Constant  Value=7
  Constant4 : Constant  Value=Vi
  Constant5 : Constant  Value=10
  Divide4 : Product  Inputs=*/
  Gain21 : Gain  Gain=18
  Gain22 : Gain  Gain=p1
  Gain23 : Gain  Gain=p2
  Gain24 : Gain  Gain=p1
  Gain25 : Gain  Gain=p3
  Gain26 : Gain  Gain=n
  Glucosa basal  4 : Constant  Value=7
  Gráfica glucosa 4 : Scope  NumInputPorts=2
  Gráfica insulina 4 : Scope  NumInputPorts=2
  Gráfica insulina activa4 : Scope
  Insulina basal      4 : Constant  Value=10
  Insulina basal    4 : Constant  Value=10
  Integrator10 : Integrator  InitialConditionSource=external
  Integrator11 : Integrator  InitialConditionSource=external  InitialCondition=7
  Integrator12 : Integrator
  Product8 : Product
  Sum{24,26..28,31} (5 alike) : Sum  Inputs=|+-
  Sum25 : Sum  Inputs=|++
  sin ret : Gain  Gain=18
  Out1 : Outport
  Out2 : Outport  Port=2
  wires:
  Gain26/1 -> Sum28/2
  Glucosa basal  4/1 -> Gain22/1, Gain21/1
  D/1 -> Sum24/1
  Gain21/1 -> Gráfica glucosa 4/2  "glucosa basal"
  Integrator11/1 -> sin ret/1, Out2/1, Gain24/1, Product8/1  "G(t)"
  Integrator12/1 -> Product8/2, Gain23/1, Gráfica insulina activa4/1  "X(t)"
  Gain25/1 -> Sum26/1
  Integrator10/1 -> Out1/1, Gráfica insulina 4/1, Sum31/1, Gain26/1  "I(t)"
  Constant5/1 -> Integrator10/2
  Sum31/1 -> Gain25/1
  Sum26/1 -> Integrator12/1
  Gain23/1 -> Sum26/2
  Sum28/1 -> Integrator10/1
  Sum24/1 -> Sum27/1
  Sum25/1 -> Integrator11/1
  Gain24/1 -> Sum24/2
  Insulina basal      4/1 -> Gráfica insulina 4/2
  Sum27/1 -> Sum25/1
  Insulina basal    4/1 -> Sum31/2
  Divide4/1 -> Sum28/1
  Gain22/1 -> Sum25/2
  Product8/1 -> Sum27/2
  Constant4/1 -> Divide4/2
  Constant/1 -> Integrator11/2
  Controlador/1 -> Divide4/1
  sin ret/1 -> Gráfica glucosa 4/1

== system EstudioReguladores/Subsystem12/Subsystem11 ==
  Controlador : Inport
  D : Inport  Port=2
  Constant : Constant  Value=7
  Constant4 : Constant  Value=Vi
  Constant5 : Constant  Value=10
  Divide4 : Product  Inputs=*/
  Gain21 : Gain  Gain=18
  Gain22 : Gain  Gain=p1
  Gain23 : Gain  Gain=p2
  Gain24 : Gain  Gain=p1
  Gain25 : Gain  Gain=p3
  Gain26 : Gain  Gain=n
  Glucosa basal  4 : Constant  Value=7
  Gráfica glucosa 4 : Scope  NumInputPorts=2
  Gráfica insulina 4 : Scope  NumInputPorts=2
  Gráfica insulina activa4 : Scope
  Insulina basal      4 : Constant  Value=10
  Insulina basal    4 : Constant  Value=10
  Integrator10 : Integrator  InitialConditionSource=external
  Integrator11 : Integrator  InitialConditionSource=external  InitialCondition=7
  Integrator12 : Integrator
  Product8 : Product
  Sum{24,26..28,31} (5 alike) : Sum  Inputs=|+-
  Sum25 : Sum  Inputs=|++
  sin ret : Gain  Gain=18
  Out1 : Outport
  Out2 : Outport  Port=2
  wires:
  Gain26/1 -> Sum28/2
  Glucosa basal  4/1 -> Gain22/1, Gain21/1
  D/1 -> Sum24/1
  Gain21/1 -> Gráfica glucosa 4/2  "glucosa basal"
  Integrator11/1 -> sin ret/1, Out2/1, Gain24/1, Product8/1  "G(t)"
  Integrator12/1 -> Product8/2, Gain23/1, Gráfica insulina activa4/1  "X(t)"
  Gain25/1 -> Sum26/1
  Integrator10/1 -> Out1/1, Gráfica insulina 4/1, Sum31/1, Gain26/1  "I(t)"
  Constant5/1 -> Integrator10/2
  Sum31/1 -> Gain25/1
  Sum26/1 -> Integrator12/1
  Gain23/1 -> Sum26/2
  Sum28/1 -> Integrator10/1
  Sum24/1 -> Sum27/1
  Sum25/1 -> Integrator11/1
  Gain24/1 -> Sum24/2
  Insulina basal      4/1 -> Gráfica insulina 4/2
  Sum27/1 -> Sum25/1
  Insulina basal    4/1 -> Sum31/2
  Divide4/1 -> Sum28/1
  Gain22/1 -> Sum25/2
  Product8/1 -> Sum27/2
  Constant4/1 -> Divide4/2
  Constant/1 -> Integrator11/2
  Controlador/1 -> Divide4/1
  sin ret/1 -> Gráfica glucosa 4/1

== system EstudioReguladores/Subsystem12/Subsystem12 ==
  Controlador : Inport
  D : Inport  Port=2
  Constant : Constant  Value=7
  Constant4 : Constant  Value=Vi
  Constant5 : Constant  Value=10
  Divide4 : Product  Inputs=*/
  Gain21 : Gain  Gain=18
  Gain22 : Gain  Gain=p1
  Gain23 : Gain  Gain=p2
  Gain24 : Gain  Gain=p1
  Gain25 : Gain  Gain=p3
  Gain26 : Gain  Gain=n
  Glucosa basal  4 : Constant  Value=7
  Gráfica glucosa 4 : Scope  NumInputPorts=2
  Gráfica insulina 4 : Scope  NumInputPorts=2
  Gráfica insulina activa4 : Scope
  Insulina basal      4 : Constant  Value=10
  Insulina basal    4 : Constant  Value=10
  Integrator10 : Integrator  InitialConditionSource=external
  Integrator11 : Integrator  InitialConditionSource=external  InitialCondition=7
  Integrator12 : Integrator
  Product8 : Product
  Sum{24,26..28,31} (5 alike) : Sum  Inputs=|+-
  Sum25 : Sum  Inputs=|++
  sin ret : Gain  Gain=18
  Out1 : Outport
  Out2 : Outport  Port=2
  wires:
  Gain26/1 -> Sum28/2
  Glucosa basal  4/1 -> Gain22/1, Gain21/1
  D/1 -> Sum24/1
  Gain21/1 -> Gráfica glucosa 4/2  "glucosa basal"
  Integrator11/1 -> sin ret/1, Out2/1, Gain24/1, Product8/1  "G(t)"
  Integrator12/1 -> Product8/2, Gain23/1, Gráfica insulina activa4/1  "X(t)"
  Gain25/1 -> Sum26/1
  Integrator10/1 -> Out1/1, Gráfica insulina 4/1, Sum31/1, Gain26/1  "I(t)"
  Constant5/1 -> Integrator10/2
  Sum31/1 -> Gain25/1
  Sum26/1 -> Integrator12/1
  Gain23/1 -> Sum26/2
  Sum28/1 -> Integrator10/1
  Sum24/1 -> Sum27/1
  Sum25/1 -> Integrator11/1
  Gain24/1 -> Sum24/2
  Insulina basal      4/1 -> Gráfica insulina 4/2
  Sum27/1 -> Sum25/1
  Insulina basal    4/1 -> Sum31/2
  Divide4/1 -> Sum28/1
  Gain22/1 -> Sum25/2
  Product8/1 -> Sum27/2
  Constant4/1 -> Divide4/2
  Constant/1 -> Integrator11/2
  Controlador/1 -> Divide4/1
  sin ret/1 -> Gráfica glucosa 4/1

== system EstudioReguladores/Subsystem12/Subsystem13 ==
  Controlador : Inport
  D : Inport  Port=2
  Constant : Constant  Value=7
  Constant4 : Constant  Value=Vi
  Constant5 : Constant  Value=10
  Divide4 : Product  Inputs=*/
  Gain21 : Gain  Gain=18
  Gain22 : Gain  Gain=p1
  Gain23 : Gain  Gain=p2
  Gain24 : Gain  Gain=p1
  Gain25 : Gain  Gain=p3
  Gain26 : Gain  Gain=n
  Glucosa basal  4 : Constant  Value=7
  Gráfica glucosa 4 : Scope  NumInputPorts=2
  Gráfica insulina 4 : Scope  NumInputPorts=2
  Gráfica insulina activa4 : Scope
  Insulina basal      4 : Constant  Value=10
  Insulina basal    4 : Constant  Value=10
  Integrator10 : Integrator  InitialConditionSource=external
  Integrator11 : Integrator  InitialConditionSource=external  InitialCondition=7
  Integrator12 : Integrator
  Product8 : Product
  Sum{24,26..28,31} (5 alike) : Sum  Inputs=|+-
  Sum25 : Sum  Inputs=|++
  sin ret : Gain  Gain=18
  Out1 : Outport
  Out2 : Outport  Port=2
  wires:
  Gain26/1 -> Sum28/2
  Glucosa basal  4/1 -> Gain22/1, Gain21/1
  D/1 -> Sum24/1
  Gain21/1 -> Gráfica glucosa 4/2  "glucosa basal"
  Integrator11/1 -> sin ret/1, Out2/1, Gain24/1, Product8/1  "G(t)"
  Integrator12/1 -> Product8/2, Gain23/1, Gráfica insulina activa4/1  "X(t)"
  Gain25/1 -> Sum26/1
  Integrator10/1 -> Out1/1, Gráfica insulina 4/1, Sum31/1, Gain26/1  "I(t)"
  Constant5/1 -> Integrator10/2
  Sum31/1 -> Gain25/1
  Sum26/1 -> Integrator12/1
  Gain23/1 -> Sum26/2
  Sum28/1 -> Integrator10/1
  Sum24/1 -> Sum27/1
  Sum25/1 -> Integrator11/1
  Gain24/1 -> Sum24/2
  Insulina basal      4/1 -> Gráfica insulina 4/2
  Sum27/1 -> Sum25/1
  Insulina basal    4/1 -> Sum31/2
  Divide4/1 -> Sum28/1
  Gain22/1 -> Sum25/2
  Product8/1 -> Sum27/2
  Constant4/1 -> Divide4/2
  Constant/1 -> Integrator11/2
  Controlador/1 -> Divide4/1
  sin ret/1 -> Gráfica glucosa 4/1

== system EstudioReguladores/Subsystem13/Subsystem10 ==
  Controlador : Inport
  D : Inport  Port=2
  Constant : Constant  Value=7
  Constant4 : Constant  Value=Vi
  Constant5 : Constant  Value=10
  Divide4 : Product  Inputs=*/
  Gain21 : Gain  Gain=18
  Gain22 : Gain  Gain=p1
  Gain23 : Gain  Gain=p2
  Gain24 : Gain  Gain=p1
  Gain25 : Gain  Gain=p3
  Gain26 : Gain  Gain=n
  Glucosa basal  4 : Constant  Value=7
  Gráfica glucosa 4 : Scope  NumInputPorts=2
  Gráfica insulina 4 : Scope  NumInputPorts=2
  Gráfica insulina activa4 : Scope
  Insulina basal      4 : Constant  Value=10
  Insulina basal    4 : Constant  Value=10
  Integrator10 : Integrator  InitialConditionSource=external
  Integrator11 : Integrator  InitialConditionSource=external  InitialCondition=7
  Integrator12 : Integrator
  Product8 : Product
  Sum{24,26..28,31} (5 alike) : Sum  Inputs=|+-
  Sum25 : Sum  Inputs=|++
  sin ret : Gain  Gain=18
  Out1 : Outport
  Out2 : Outport  Port=2
  wires:
  Gain26/1 -> Sum28/2
  Glucosa basal  4/1 -> Gain22/1, Gain21/1
  D/1 -> Sum24/1
  Gain21/1 -> Gráfica glucosa 4/2  "glucosa basal"
  Integrator11/1 -> sin ret/1, Out2/1, Gain24/1, Product8/1  "G(t)"
  Integrator12/1 -> Product8/2, Gain23/1, Gráfica insulina activa4/1  "X(t)"
  Gain25/1 -> Sum26/1
  Integrator10/1 -> Out1/1, Gráfica insulina 4/1, Sum31/1, Gain26/1  "I(t)"
  Constant5/1 -> Integrator10/2
  Sum31/1 -> Gain25/1
  Sum26/1 -> Integrator12/1
  Gain23/1 -> Sum26/2
  Sum28/1 -> Integrator10/1
  Sum24/1 -> Sum27/1
  Sum25/1 -> Integrator11/1
  Gain24/1 -> Sum24/2
  Insulina basal      4/1 -> Gráfica insulina 4/2
  Sum27/1 -> Sum25/1
  Insulina basal    4/1 -> Sum31/2
  Divide4/1 -> Sum28/1
  Gain22/1 -> Sum25/2
  Product8/1 -> Sum27/2
  Constant4/1 -> Divide4/2
  Constant/1 -> Integrator11/2
  Controlador/1 -> Divide4/1
  sin ret/1 -> Gráfica glucosa 4/1

== system EstudioReguladores/Subsystem13/Subsystem11 ==
  Controlador : Inport
  D : Inport  Port=2
  Constant : Constant  Value=7
  Constant4 : Constant  Value=Vi
  Constant5 : Constant  Value=10
  Divide4 : Product  Inputs=*/
  Gain21 : Gain  Gain=18
  Gain22 : Gain  Gain=p1
  Gain23 : Gain  Gain=p2
  Gain24 : Gain  Gain=p1
  Gain25 : Gain  Gain=p3
  Gain26 : Gain  Gain=n
  Glucosa basal  4 : Constant  Value=7
  Gráfica glucosa 4 : Scope  NumInputPorts=2
  Gráfica insulina 4 : Scope  NumInputPorts=2
  Gráfica insulina activa4 : Scope
  Insulina basal      4 : Constant  Value=10
  Insulina basal    4 : Constant  Value=10
  Integrator10 : Integrator  InitialConditionSource=external
  Integrator11 : Integrator  InitialConditionSource=external  InitialCondition=7
  Integrator12 : Integrator
  Product8 : Product
  Sum{24,26..28,31} (5 alike) : Sum  Inputs=|+-
  Sum25 : Sum  Inputs=|++
  sin ret : Gain  Gain=18
  Out1 : Outport
  Out2 : Outport  Port=2
  wires:
  Gain26/1 -> Sum28/2
  Glucosa basal  4/1 -> Gain22/1, Gain21/1
  D/1 -> Sum24/1
  Gain21/1 -> Gráfica glucosa 4/2  "glucosa basal"
  Integrator11/1 -> sin ret/1, Out2/1, Gain24/1, Product8/1  "G(t)"
  Integrator12/1 -> Product8/2, Gain23/1, Gráfica insulina activa4/1  "X(t)"
  Gain25/1 -> Sum26/1
  Integrator10/1 -> Out1/1, Gráfica insulina 4/1, Sum31/1, Gain26/1  "I(t)"
  Constant5/1 -> Integrator10/2
  Sum31/1 -> Gain25/1
  Sum26/1 -> Integrator12/1
  Gain23/1 -> Sum26/2
  Sum28/1 -> Integrator10/1
  Sum24/1 -> Sum27/1
  Sum25/1 -> Integrator11/1
  Gain24/1 -> Sum24/2
  Insulina basal      4/1 -> Gráfica insulina 4/2
  Sum27/1 -> Sum25/1
  Insulina basal    4/1 -> Sum31/2
  Divide4/1 -> Sum28/1
  Gain22/1 -> Sum25/2
  Product8/1 -> Sum27/2
  Constant4/1 -> Divide4/2
  Constant/1 -> Integrator11/2
  Controlador/1 -> Divide4/1
  sin ret/1 -> Gráfica glucosa 4/1

== system EstudioReguladores/Subsystem13/Subsystem12 ==
  Controlador : Inport
  D : Inport  Port=2
  Constant : Constant  Value=7
  Constant4 : Constant  Value=Vi
  Constant5 : Constant  Value=10
  Divide4 : Product  Inputs=*/
  Gain21 : Gain  Gain=18
  Gain22 : Gain  Gain=p1
  Gain23 : Gain  Gain=p2
  Gain24 : Gain  Gain=p1
  Gain25 : Gain  Gain=p3
  Gain26 : Gain  Gain=n
  Glucosa basal  4 : Constant  Value=7
  Gráfica glucosa 4 : Scope  NumInputPorts=2
  Gráfica insulina 4 : Scope  NumInputPorts=2
  Gráfica insulina activa4 : Scope
  Insulina basal      4 : Constant  Value=10
  Insulina basal    4 : Constant  Value=10
  Integrator10 : Integrator  InitialConditionSource=external
  Integrator11 : Integrator  InitialConditionSource=external  InitialCondition=7
  Integrator12 : Integrator
  Product8 : Product
  Sum{24,26..28,31} (5 alike) : Sum  Inputs=|+-
  Sum25 : Sum  Inputs=|++
  sin ret : Gain  Gain=18
  Out1 : Outport
  Out2 : Outport  Port=2
  wires:
  Gain26/1 -> Sum28/2
  Glucosa basal  4/1 -> Gain22/1, Gain21/1
  D/1 -> Sum24/1
  Gain21/1 -> Gráfica glucosa 4/2  "glucosa basal"
  Integrator11/1 -> sin ret/1, Out2/1, Gain24/1, Product8/1  "G(t)"
  Integrator12/1 -> Product8/2, Gain23/1, Gráfica insulina activa4/1  "X(t)"
  Gain25/1 -> Sum26/1
  Integrator10/1 -> Out1/1, Gráfica insulina 4/1, Sum31/1, Gain26/1  "I(t)"
  Constant5/1 -> Integrator10/2
  Sum31/1 -> Gain25/1
  Sum26/1 -> Integrator12/1
  Gain23/1 -> Sum26/2
  Sum28/1 -> Integrator10/1
  Sum24/1 -> Sum27/1
  Sum25/1 -> Integrator11/1
  Gain24/1 -> Sum24/2
  Insulina basal      4/1 -> Gráfica insulina 4/2
  Sum27/1 -> Sum25/1
  Insulina basal    4/1 -> Sum31/2
  Divide4/1 -> Sum28/1
  Gain22/1 -> Sum25/2
  Product8/1 -> Sum27/2
  Constant4/1 -> Divide4/2
  Constant/1 -> Integrator11/2
  Controlador/1 -> Divide4/1
  sin ret/1 -> Gráfica glucosa 4/1

== system EstudioReguladores/Subsystem13/Subsystem13 ==
  Controlador : Inport
  D : Inport  Port=2
  Constant : Constant  Value=7
  Constant4 : Constant  Value=Vi
  Constant5 : Constant  Value=10
  Divide4 : Product  Inputs=*/
  Gain21 : Gain  Gain=18
  Gain22 : Gain  Gain=p1
  Gain23 : Gain  Gain=p2
  Gain24 : Gain  Gain=p1
  Gain25 : Gain  Gain=p3
  Gain26 : Gain  Gain=n
  Glucosa basal  4 : Constant  Value=7
  Gráfica glucosa 4 : Scope  NumInputPorts=2
  Gráfica insulina 4 : Scope  NumInputPorts=2
  Gráfica insulina activa4 : Scope
  Insulina basal      4 : Constant  Value=10
  Insulina basal    4 : Constant  Value=10
  Integrator10 : Integrator  InitialConditionSource=external
  Integrator11 : Integrator  InitialConditionSource=external  InitialCondition=7
  Integrator12 : Integrator
  Product8 : Product
  Sum{24,26..28,31} (5 alike) : Sum  Inputs=|+-
  Sum25 : Sum  Inputs=|++
  sin ret : Gain  Gain=18
  Out1 : Outport
  Out2 : Outport  Port=2
  wires:
  Gain26/1 -> Sum28/2
  Glucosa basal  4/1 -> Gain22/1, Gain21/1
  D/1 -> Sum24/1
  Gain21/1 -> Gráfica glucosa 4/2  "glucosa basal"
  Integrator11/1 -> sin ret/1, Out2/1, Gain24/1, Product8/1  "G(t)"
  Integrator12/1 -> Product8/2, Gain23/1, Gráfica insulina activa4/1  "X(t)"
  Gain25/1 -> Sum26/1
  Integrator10/1 -> Out1/1, Gráfica insulina 4/1, Sum31/1, Gain26/1  "I(t)"
  Constant5/1 -> Integrator10/2
  Sum31/1 -> Gain25/1
  Sum26/1 -> Integrator12/1
  Gain23/1 -> Sum26/2
  Sum28/1 -> Integrator10/1
  Sum24/1 -> Sum27/1
  Sum25/1 -> Integrator11/1
  Gain24/1 -> Sum24/2
  Insulina basal      4/1 -> Gráfica insulina 4/2
  Sum27/1 -> Sum25/1
  Insulina basal    4/1 -> Sum31/2
  Divide4/1 -> Sum28/1
  Gain22/1 -> Sum25/2
  Product8/1 -> Sum27/2
  Constant4/1 -> Divide4/2
  Constant/1 -> Integrator11/2
  Controlador/1 -> Divide4/1
  sin ret/1 -> Gráfica glucosa 4/1

== system EstudioReguladores/Subsystem14/Subsystem10 ==
  Controlador : Inport
  D : Inport  Port=2
  Constant : Constant  Value=7
  Constant4 : Constant  Value=Vi
  Constant5 : Constant  Value=10
  Divide4 : Product  Inputs=*/
  Gain21 : Gain  Gain=18
  Gain22 : Gain  Gain=p1
  Gain23 : Gain  Gain=p2
  Gain24 : Gain  Gain=p1
  Gain25 : Gain  Gain=p3
  Gain26 : Gain  Gain=n
  Glucosa basal  4 : Constant  Value=7
  Gráfica glucosa 4 : Scope  NumInputPorts=2
  Gráfica insulina 4 : Scope  NumInputPorts=2
  Gráfica insulina activa4 : Scope
  Insulina basal      4 : Constant  Value=10
  Insulina basal    4 : Constant  Value=10
  Integrator10 : Integrator  InitialConditionSource=external
  Integrator11 : Integrator  InitialConditionSource=external  InitialCondition=7
  Integrator12 : Integrator
  Product8 : Product
  Sum{24,26..28,31} (5 alike) : Sum  Inputs=|+-
  Sum25 : Sum  Inputs=|++
  sin ret : Gain  Gain=18
  Out1 : Outport
  Out2 : Outport  Port=2
  wires:
  Gain26/1 -> Sum28/2
  Glucosa basal  4/1 -> Gain22/1, Gain21/1
  D/1 -> Sum24/1
  Gain21/1 -> Gráfica glucosa 4/2  "glucosa basal"
  Integrator11/1 -> sin ret/1, Out2/1, Gain24/1, Product8/1  "G(t)"
  Integrator12/1 -> Product8/2, Gain23/1, Gráfica insulina activa4/1  "X(t)"
  Gain25/1 -> Sum26/1
  Integrator10/1 -> Out1/1, Gráfica insulina 4/1, Sum31/1, Gain26/1  "I(t)"
  Constant5/1 -> Integrator10/2
  Sum31/1 -> Gain25/1
  Sum26/1 -> Integrator12/1
  Gain23/1 -> Sum26/2
  Sum28/1 -> Integrator10/1
  Sum24/1 -> Sum27/1
  Sum25/1 -> Integrator11/1
  Gain24/1 -> Sum24/2
  Insulina basal      4/1 -> Gráfica insulina 4/2
  Sum27/1 -> Sum25/1
  Insulina basal    4/1 -> Sum31/2
  Divide4/1 -> Sum28/1
  Gain22/1 -> Sum25/2
  Product8/1 -> Sum27/2
  Constant4/1 -> Divide4/2
  Constant/1 -> Integrator11/2
  Controlador/1 -> Divide4/1
  sin ret/1 -> Gráfica glucosa 4/1
